simulink model "Global_system_simulation"  (R2014a)
settings: Solver=ode45  StartTime=0.0  StopTime=12.2474  FixedStep=0.02  RelTol=1e-3
settings Model: Creator=Eric  LastModifiedBy=Administrator
settings DataIOCC: InspectSignalLogs=on

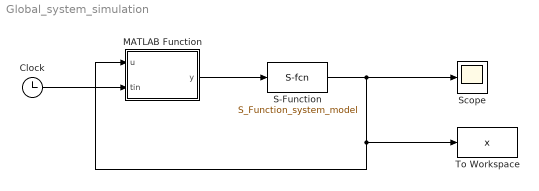
== system Global_system_simulation ==
  Clock : Clock
  MATLAB Function : MATLAB Function  TreatAsAtomicUnit=on
  S-Function : S-Function  FunctionName=S_Function_system_model  Parameters=[23.50;0;0.0448;0;20]  EnableBusSupport=off
  Scope : Scope
      settings: YMin=-2.5  YMax=30
  To Workspace : ToWorkspace  VariableName=x  SaveFormat=Timeseries  SampleTime=-1
  wires:
  Clock/1 -> MATLAB Function/2(tin)
  MATLAB Function/1(y) -> S-Function/1
  S-Function/1 -> To Workspace/1, MATLAB Function/1(u), Scope/1

== matlab function Global_system_simulation/MATLAB Function ==
  data: u input; y output; tin input
%function y = fcn(u, tin)
%控制器部分：求控制器输出（虚拟升降舵 油门）  
function y = fcn(u,tin)


y = [0;0];       %开环系统过渡过程测试


end
